simulink model "SimV4"  (R2024b)
settings: Solver=VariableStepAuto  StartTime=0.0  StopTime=30  RelTol=1e-3
model workspace (MAT data in the model file):
  Sig = Simulink.Signal
  Sig.Dimensions = -1
  Sig.DimensionsMode = 'auto'
  Sig.Complexity = 'auto'
  Sig.SampleTime = -1
  Sig.SamplingMode = 'auto'
  Sig.DataType = 'auto'
values from neighbouring files (symbols this model uses):
  CanaryAmplitude = 0.25    [ConfigData.sldd]
  CanaryCarrierFrequency = 20000.0    [ConfigData.sldd]
  CanaryDataRate = 100.0    [ConfigData.sldd]
  DataAmplitude = 0.1    [ConfigData.sldd]
  PreConvolveDownsample = 32.0    [ConfigData.sldd]
  SampleRate = 48000.0    [ConfigData.sldd]
  WalshCodeIndex = 9.0 3.0    [ConfigData.sldd]
undefined symbols (not defined in the file or in its folder): magnitude, WalshCodeCache
libraries: dspfdesign x7, simulink x3, audiosources x2, dspstat3 x2, dspsigops x2, commseqgen3 x2, commchan3 x1, dspsnks4 x1
settings Model: DataDictionary=ConfigData.sldd  SimulationMode=accelerator  PauseTimes=4.5  PacingRate=0.007100  Creator=calum  LastModifiedBy=calum
settings SolverCC: AllowMultiTaskInputOutput=on
settings OptimizationCC: StateBitsets=on  DataBitsets=on  SimCompilerOptimization=on  AccelVerboseBuild=on
settings DebuggingCC: IntegerOverflowMsg=none  IntegerSaturationMsg=none
settings HardwareCC: ProdBitPerLong=64  ProdHWDeviceType=Intel->x86-64 (Linux 64)
settings ModelReferenceCC: UpdateModelReferenceTargets=IfOutOfDate  EnableParallelModelReferenceBuilds=on  ParallelModelReferenceMATLABWorkerInit=Copy Base Workspace
settings SFSimCC: SimCtrlC=off  SimHardwareAcceleration=native
settings RTWCC: GenerateReport=on  Toolchain=GNU gcc/g++ | gmake (64-bit Linux)  BuildConfiguration=Specify  LaunchReport=on
settings GRTTargetCC: OptimizeReductions=on

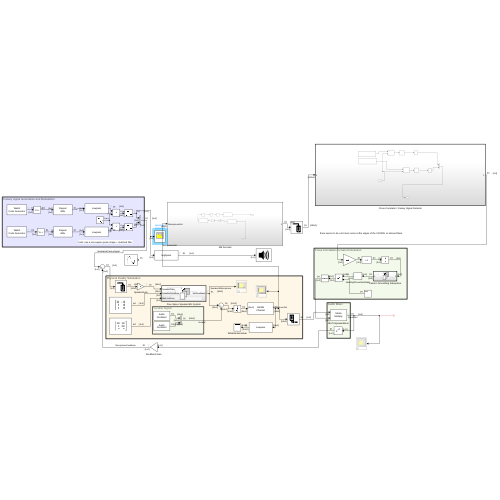
[thumbnail: Simulink's stored preview of the top-level diagram]
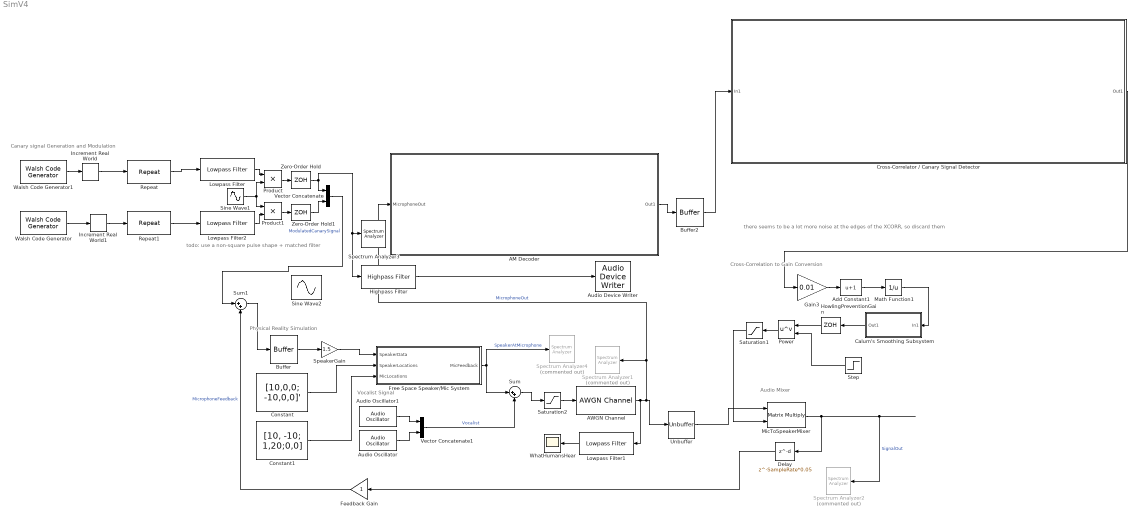
== system SimV4 ==
  note: Canary signal Generation and Modulation
  note: Audio Mixer
  note: Physical Reality Simulation
  note: Vocalist Signal
  note: Cross-Correlation to Gain Conversion
  note: there seems to be a lot more noise at the edges of the XCORR, so discard them
  note: todo: use a non-square pulse shape + matched filter
  "AM Decoder " : Subsystem  Latency=2
  AWGN Channel : commchan3/AWGN Channel  LegacyMode=off  NoiseMethod="Signal to noise ratio  (SNR)"  noiseMode="Signal to noise ratio  (SNR)"  EbNo=10  EsNo=10  SNR=60  BitsPerSymbol=1  SignalPower=1  SamplesPerSymbol=1  SymbolPeriod=1  VarianceSource=Parameter  Variance=1  RandomStream=Global stream  Seed=67  SimulateUsing=Code generation
  Add Constant1 : Bias  Bias=1  SaturateOnIntegerOverflow=off
  Audio Device Writer : dspsnks4/Audio Device Writer  Driver=ALSA  Device=HDA Intel PCH: ALC3254 Analog (hw:0,0)  InheritSampleRate=off  SampleRate=SampleRate  BitDepth=32-bit float  BufferSize=4096  NumBuffers=10  DefaultOutputChannelMapping=on  OutputChannelMapping=1:2  OutputNumUnderrunSamples=off  DriverIdx=8  DeviceWarnFlag=''
  Audio Oscillator : audiosources/Audio Oscillator  FrequencyPort=off  Frequency=200  AmplitudePort=off  Amplitude=DataAmplitude  DCOffsetPort=off  DCOffset=0  PhaseOffset=0  WidthPort=off  Width=1  DutyCyclePort=off  DutyCycle=0.5  SampsPerFrame=64  Fs=SampleRate  OutputDataType=double  SimulateUsing=Code generation
      settings: SignalType=sine
  Audio Oscillator1 : audiosources/Audio Oscillator  FrequencyPort=off  Frequency=400  AmplitudePort=off  Amplitude=DataAmplitude  DCOffsetPort=off  DCOffset=0  PhaseOffset=0  WidthPort=off  Width=1  DutyCyclePort=off  DutyCycle=0.5  SampsPerFrame=64  Fs=SampleRate  OutputDataType=double  SimulateUsing=Code generation
      settings: SignalType=sine
  Buffer : Buffer  OutputFrames=off
  Buffer2 : Buffer  N=ceil(SampleRate/32/CanaryDataRate*32)+10  V=ceil(SampleRate/32/CanaryDataRate*32)+2  OutputFrames=off
  Calum's Smoothing Subsystem : Subsystem  TreatAsAtomicUnit=on
  Constant : Constant  Value="[10,0,0;  -10,0,0]'"
  Constant1 : Constant  Value=[10, -10; 1,20;0,0]
  "Cross-Correlator / Canary Signal Detector " : Subsystem  TreatAsAtomicUnit=on
  Delay : Delay  DelayLength=SampleRate*0.05  InitialCondition=0
  Feedback Gain : Gain
  Free Space Speaker/Mic System : Subsystem  TreatAsAtomicUnit=on
  Gain3 : Gain  Gain=0.01
  Highpass Filter : dspfdesign/Highpass Filter  FilterType=FIR  DesignForMinimumOrder=on  FilterOrder=50  StopbandFrequency=CanaryCarrierFrequency-1000  PassbandFrequency=CanaryCarrierFrequency  StopbandAttenuation=80  PassbandRipple=0.1  SampleRateMode=Specify on dialog  SampleRate=SampleRate  SimulateUsing=Code generation  roundingMode=Floor  coeffsDataTypeStr=fixdt(1,16)
  HowlingPreventionGain : ZeroOrderHold  SampleTime=1/(CanaryDataRate)
  Increment Real World : simulink/Additional Math & Discrete/Additional Math: Increment - Decrement/Increment Real World
  Increment Real World1 : simulink/Additional Math & Discrete/Additional Math: Increment - Decrement/Increment Real World
  Lowpass Filter : dspfdesign/Lowpass Filter  FilterType=IIR  DesignForMinimumOrder=on  FilterOrder=50  PassbandFrequency=CanaryDataRate*2  StopbandFrequency=CanaryDataRate*10  PassbandRipple=0.5  StopbandAttenuation=80  SampleRateMode=Specify on dialog  SampleRate=SampleRate  SimulateUsing=Code generation  roundingMode=Floor  coeffsDataTypeStr=fixdt(1,16)
  Lowpass Filter1 : dspfdesign/Lowpass Filter  FilterType=FIR  DesignForMinimumOrder=on  FilterOrder=50  PassbandFrequency=CanaryCarrierFrequency-8000  StopbandFrequency=CanaryCarrierFrequency-1000  PassbandRipple=0.1  StopbandAttenuation=80  SampleRateMode=Specify on dialog  SampleRate=SampleRate  SimulateUsing=Code generation  roundingMode=Floor  coeffsDataTypeStr=fixdt(1,16)
  Lowpass Filter2 : dspfdesign/Lowpass Filter  FilterType=IIR  DesignForMinimumOrder=on  FilterOrder=50  PassbandFrequency=CanaryDataRate*2  StopbandFrequency=CanaryDataRate*10  PassbandRipple=0.5  StopbandAttenuation=80  SampleRateMode=Specify on dialog  SampleRate=SampleRate  SimulateUsing=Code generation  roundingMode=Floor  coeffsDataTypeStr=fixdt(1,16)
  Math Function1 : Math  Operator=reciprocal
  MicToSpeakerMixer : Product  Multiplication=Matrix(*)
  Power : Math  Operator=pow
  Product : Product
  Product1 : Product
  Repeat : dspsigops/Repeat  FactorSource=Dialog parameter  N=SampleRate/CanaryDataRate  Nmax=16  InputProcessing=Columns as channels (frame based)  RateOptions=Allow multirate processing  ic=0  mode=Unused parameter value
      settings: LibrarySourceBlock=commsequence2/Repeat
  Repeat1 : dspsigops/Repeat  FactorSource=Dialog parameter  N=SampleRate/CanaryDataRate  Nmax=16  InputProcessing=Columns as channels (frame based)  RateOptions=Allow multirate processing  ic=0  mode=Unused parameter value
      settings: LibrarySourceBlock=commsequence2/Repeat
  Saturation1 : Saturate  UpperLimit=1  LowerLimit=0
  Saturation2 : Saturate  UpperLimit=1000  LowerLimit=-1000
  Sine Wave1 : Sin  Amplitude=CanaryAmplitude  Frequency=2*pi*CanaryCarrierFrequency  SampleTime=0
  Sine Wave2 : Sin  Frequency=2*pi*(CanaryCarrierFrequency-1000)  SampleTime=1/SampleRate
  SpeakerGain : Gain  Gain=1.5
  Spectrum Analyzer1 : SpectrumAnalyzer  Commented=on  WindowPosition=[1.000000,38.000000,1920.000000,1003.000000,]  ScopeFrameLocation=window  SampleRateSource=Property  SampleRate=SampleRate  PlotAsTwoSidedSpectrum=off  FrequencyScale=Log  FrequencySpan=Start and stop frequencies  StartFrequency=20  StopFrequency=20e3  YLimits=[-78.74086897,62.76889366]
  Spectrum Analyzer2 : SpectrumAnalyzer  Commented=on  WindowPosition=[1.000000,38.000000,1920.000000,1003.000000,]  ScopeFrameLocation=window  SampleRateSource=Property  SampleRate=SampleRate  PlotAsTwoSidedSpectrum=off  FrequencyScale=Log  FrequencySpan=Start and stop frequencies  StartFrequency=20  StopFrequency=20e3  YLimits=[-81.26361088,68.62221432]
  Spectrum Analyzer3 : SpectrumAnalyzer  WindowPosition=[1.000000,1.000000,1920.000000,1003.000000,]  Visible=on  ScopeFrameLocation=window  Method=Welch  SampleRateSource=Property  SampleRate=SampleRate  PlotAsTwoSidedSpectrum=off  FrequencyScale=Log  FrequencySpan=Start and stop frequencies  StartFrequency=20  StopFrequency=SampleRate/2  YLimits=[-147.26950534,47.28576259]  SelectedToolstripTab=spectrumAnalyzerToolstrip.estimationTab
  Spectrum Analyzer4 : SpectrumAnalyzer  Commented=on  WindowPosition=[1.000000,38.000000,1920.000000,1003.000000,]  ScopeFrameLocation=window  ViewType=Spectrum and spectrogram  SampleRateSource=Property  SampleRate=SampleRate  PlotAsTwoSidedSpectrum=off  FrequencyScale=Log  FrequencySpan=Start and stop frequencies  StartFrequency=20  StopFrequency=20e3  YLimits=[-136.03313301,69.13471038]  ColorLimits=[-136.03313301,69.13471038]
  Step : Step  Time=35  Before=5  After=0  SampleTime=1/(CanaryDataRate)
  Sum : Sum  Inputs=|++
  Sum1 : Sum  Inputs=|++
  Unbuffer : Unbuffer
  Vector Concatenate : Concatenate  Mode=Multidimensional array  ConcatenateDimension=2
  Vector Concatenate1 : Concatenate  Mode=Multidimensional array  ConcatenateDimension=2
  Walsh Code Generator : commseqgen3/Walsh Code Generator  Length=16  Index=WalshCodeIndex(2)  SampleTime=1/CanaryDataRate  SamplesPerFrame=1  OutputDataType=double  SimulateUsing=Code generation
  Walsh Code Generator1 : commseqgen3/Walsh Code Generator  Length=16  Index=WalshCodeIndex(1)  SampleTime=1/CanaryDataRate  SamplesPerFrame=1  OutputDataType=double  SimulateUsing=Code generation
  WhatHumansHear : Scope
  Zero-Order Hold : ZeroOrderHold  SampleTime=1/SampleRate
  Zero-Order Hold1 : ZeroOrderHold  SampleTime=1/SampleRate
  wires:
  Sine Wave1/1 -> Product/2, Product1/1
  Product/1 -> Zero-Order Hold/1
  Zero-Order Hold1/1 -> Vector Concatenate/2
  Product1/1 -> Zero-Order Hold1/1
  Buffer/1 -> SpeakerGain/1
  Walsh Code Generator1/1 -> Increment Real World/1
  AWGN Channel/1 -> "AM Decoder "/1(MicrophoneOut), Spectrum Analyzer1/1, Unbuffer/1, Lowpass Filter1/1  "MicrophoneOut"
  SpeakerGain/1 -> Free Space Speaker/Mic System/1(SpeakerData)
  Constant/1 -> Free Space Speaker/Mic System/2(SpeakerLocations)
  Constant1/1 -> Free Space Speaker/Mic System/3(MicLocations)
  Increment Real World/1 -> Repeat/1
  Increment Real World1/1 -> Repeat1/1
  Audio Oscillator1/1 -> Vector Concatenate1/1
  Audio Oscillator/1 -> Vector Concatenate1/2
  Add Constant1/1 -> Math Function1/1
  Gain3/1 -> Add Constant1/1
  Vector Concatenate1/1 -> Sum/2  "Vocalist"
  Free Space Speaker/Mic System/1(MicFeedback) -> Sum/1, Spectrum Analyzer4/1  "SpeakerAtMicrophone"
  Sum/1 -> Saturation2/1
  Unbuffer/1 -> MicToSpeakerMixer/1
  Math Function1/1 -> Calum's Smoothing Subsystem/1(In1)
  MicToSpeakerMixer/1 -> Spectrum Analyzer2/1, Delay/1  "SignalOut"
  Calum's Smoothing Subsystem/1(Out1) -> HowlingPreventionGain/1
  Sum1/1 -> Buffer/1
  Delay/1 -> Feedback Gain/1
  HowlingPreventionGain/1 -> Power/1
  Step/1 -> Power/2
  Vector Concatenate/1 -> Sum1/1  "ModulatedCanarySignal"
  Power/1 -> Saturation1/1
  Saturation1/1 -> MicToSpeakerMixer/2
  Saturation2/1 -> AWGN Channel/1
  Feedback Gain/1 -> Sum1/2  "MicrophoneFeedback"
  Lowpass Filter1/1 -> WhatHumansHear/1
  "AM Decoder "/1(Out1) -> Buffer2/1
  Buffer2/1 -> "Cross-Correlator / Canary Signal Detector "/1(In1)
  "Cross-Correlator / Canary Signal Detector "/1(Out1) -> Gain3/1
  Lowpass Filter/1 -> Product/1
  Walsh Code Generator/1 -> Increment Real World1/1
  Lowpass Filter2/1 -> Product1/2
  Repeat/1 -> Lowpass Filter/1
  Repeat1/1 -> Lowpass Filter2/1
  Highpass Filter/1 -> Audio Device Writer/1
  Zero-Order Hold/1 -> Vector Concatenate/1, Highpass Filter/1, Spectrum Analyzer3/1

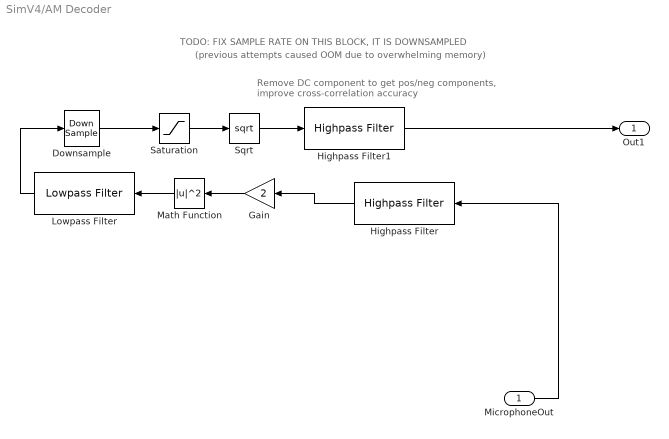
== system SimV4/AM Decoder  ==
  note: (previous attempts caused OOM due to overwhelming memory)
  note: TODO: FIX SAMPLE RATE ON THIS BLOCK, IT IS DOWNSAMPLED
  note: Remove DC component to get pos/neg components,
      | improve cross-correlation accuracy
  MicrophoneOut : Inport
  Downsample : DownSample  N=32
  Gain : Gain  Gain=2
  Highpass Filter : dspfdesign/Highpass Filter  FilterType=FIR  DesignForMinimumOrder=on  FilterOrder=50  StopbandFrequency=CanaryCarrierFrequency-20*CanaryDataRate  PassbandFrequency=CanaryCarrierFrequency-3*CanaryDataRate  StopbandAttenuation=80  PassbandRipple=2  SampleRateMode=Specify on dialog  SampleRate=SampleRate  SimulateUsing=Code generation  roundingMode=Floor  coeffsDataTypeStr=fixdt(1,16)
  Highpass Filter1 : dspfdesign/Highpass Filter  FilterType=FIR  DesignForMinimumOrder=on  FilterOrder=50  StopbandFrequency=5  PassbandFrequency=CanaryDataRate  StopbandAttenuation=80  PassbandRipple=1  SampleRateMode=Specify on dialog  SampleRate=SampleRate  SimulateUsing=Code generation  roundingMode=Floor  coeffsDataTypeStr=fixdt(1,16)
  Lowpass Filter : dspfdesign/Lowpass Filter  FilterType=FIR  DesignForMinimumOrder=on  FilterOrder=50  PassbandFrequency=CanaryDataRate*2  StopbandFrequency=CanaryDataRate*20  PassbandRipple=0.1  StopbandAttenuation=80  SampleRateMode=Specify on dialog  SampleRate=SampleRate  SimulateUsing=Code generation  roundingMode=Floor  coeffsDataTypeStr=fixdt(1,16)
  Math Function : Math  Operator=magnitude^2
  Saturation : Saturate  UpperLimit=inf  LowerLimit=0
  Sqrt : Sqrt
  Out1 : Outport
  wires:
  Gain/1 -> Math Function/1
  Highpass Filter/1 -> Gain/1
  Highpass Filter1/1 -> Out1/1
  Lowpass Filter/1 -> Downsample/1
  Math Function/1 -> Lowpass Filter/1
  Sqrt/1 -> Highpass Filter1/1
  Saturation/1 -> Sqrt/1
  Downsample/1 -> Saturation/1
  MicrophoneOut/1 -> Highpass Filter/1

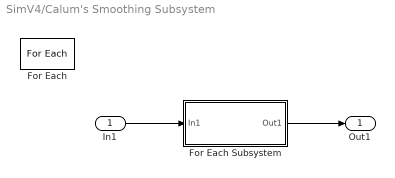
== system SimV4/Calum's Smoothing Subsystem ==
  In1 : Inport  Partition=on  PartitionDimension=1  PartitionWidth=1  PartitionOffset=0
  For Each : ForEach  DisableCoverage=on
  For Each Subsystem : Subsystem  TreatAsAtomicUnit=on
  Out1 : Outport  ConcatenationDimension=1
  wires:
  In1/1 -> For Each Subsystem/1(In1)
  For Each Subsystem/1(Out1) -> Out1/1

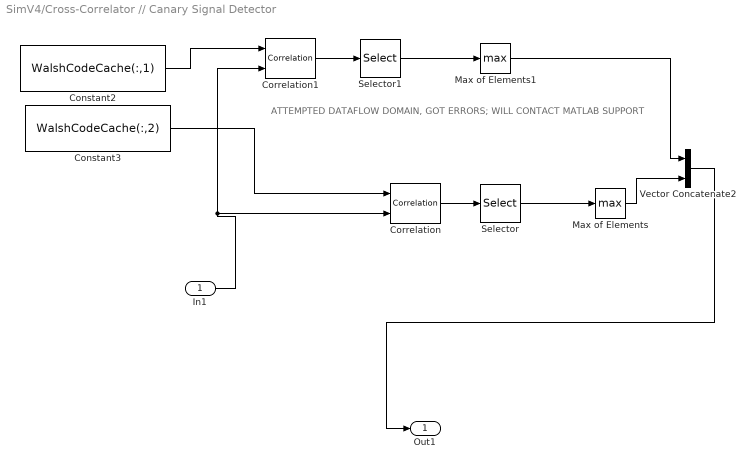
== system SimV4/Cross-Correlator // Canary Signal Detector  ==
  note: ATTEMPTED DATAFLOW DOMAIN, GOT ERRORS; WILL CONTACT MATLAB SUPPORT
  In1 : Inport
  Constant2 : Constant  Value=WalshCodeCache(:,1)  VectorParams1D=off
  Constant3 : Constant  Value=WalshCodeCache(:,2)  VectorParams1D=off
  Correlation : dspstat3/Correlation  domain=Time  roundingMode=Floor  overflowMode=off  outputDataTypeStr=Inherit: Same as accumulator  outputMin=[]  outputMax=[]  outputLastDataTypeStr=Inherit: Same as accumulator
  Correlation1 : dspstat3/Correlation  domain=Fastest  roundingMode=Floor  overflowMode=off  outputDataTypeStr=Inherit: Same as accumulator  outputMin=[]  outputMax=[]  outputLastDataTypeStr=Inherit: Same as accumulator
  Max of Elements : MinMax  Function=max  CollapseMode=Specified dimension
  Max of Elements1 : MinMax  Function=max  CollapseMode=Specified dimension
  Selector : Selector  NumberOfDimensions=2  InputPortWidth=3  IndexOptions=Index vector (dialog),Select all  Indices=[225 : 225+221],1  OutputSizes=1,1
  Selector1 : Selector  NumberOfDimensions=2  InputPortWidth=3  IndexOptions=Index vector (dialog),Select all  Indices=[225 : 225+221],1  OutputSizes=1,1
  Vector Concatenate2 : Concatenate  Mode=Multidimensional array
  Out1 : Outport
  wires:
  Constant2/1 -> Correlation1/1
  Selector/1 -> Max of Elements/1
  Constant3/1 -> Correlation/1
  Max of Elements1/1 -> Vector Concatenate2/1
  Max of Elements/1 -> Vector Concatenate2/2
  Correlation/1 -> Selector/1
  Correlation1/1 -> Selector1/1
  In1/1 -> Correlation/2, Correlation1/2
  Selector1/1 -> Max of Elements1/1
  Vector Concatenate2/1 -> Out1/1

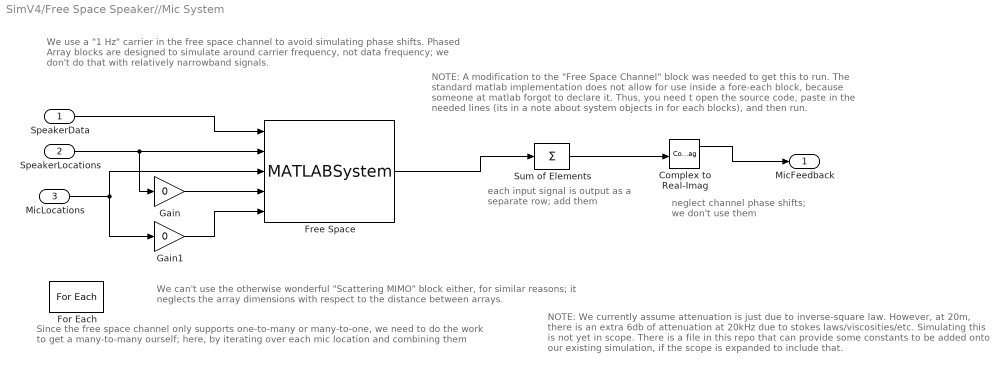
== system SimV4/Free Space Speaker//Mic System ==
  note: NOTE: We currently assume attenuation is just due to inverse-square law.
      | However, at 20m, there is an extra 6db of attenuation at 20kHz due to stokes laws/viscosities/etc.  Simulating this is not yet in scope.  There is a file in this repo that can provide some constants to be added onto our existing simulation, if the scope is expanded to include that.
  note: neglect channel phase
      | shifts; we don't use them
  note: each input signal is output as
      | a separate row; add them
  note: NOTE: A modification to the "Free Space Channel" block was needed to get
      | this to run.  The standard matlab implementation does not allow for use inside a fore-each block, because someone at matlab forgot to declare it.  Thus, you need t open the source code, paste in the needed lines (its in a note about system objects in for each blocks), and then run.
  note: Since the free space channel only supports one-to-many or many-to-one, we need to do the work to get a many-to-many ourself; here, by iterating over each mic location and combining them
  note: We can't use the otherwise wonderful "Scattering MIMO" block either, for similar reasons;
      | it neglects the array dimensions with respect to the distance between arrays.
  note: We use a "1 Hz" carrier in the free space channel to avoid simulating phase shifts.
      | Phased Array blocks are designed to simulate around carrier frequency, not data frequency; we don't do that
      | with relatively narrowband signals.
  SpeakerData : Inport
  SpeakerLocations : Inport  Port=2
  MicLocations : Inport  Port=3  Partition=on  PartitionDimension=2  PartitionWidth=1  PartitionOffset=0
  Complex to Real-Imag : ComplexToRealImag
  For Each : ForEach  DisableCoverage=on
  Free Space : MATLABSystem  System=FreeSpaceCalum  PropagationSpeed=SoundSpeed  OperatingFrequency=0.000001  TwoWayPropagation=off  SampleRateFromInputCheckbox=on  SampleRate=1e6  MaximumDistanceSource=Property  MaximumDistance=10e3  MaximumNumInputSamplesSource=Auto  MaximumNumInputSamples=100  SimulateUsing=Code generation
      settings: LibrarySourceBlock=phasedenvlib/Free Space
      mask Type: FreeSpaceCalum
      mask Display:
      | disp(['Free Space' char(10) 'Channel (Calum''s)']);
      | port_label('input',1,'X');
      | port_label('input',2,'Pos1');
      | port_label('input',3,'Pos2');
      | port_label('input',4,'Vel1');
      | port_label('input',5,'Vel2');
  Gain : Gain  Gain=0
  Gain1 : Gain  Gain=0
  Sum of Elements : Sum  Inputs=+  CollapseMode=Specified dimension  CollapseDim=2
  MicFeedback : Outport  ConcatenationDimension=2
  wires:
  SpeakerData/1 -> Free Space/1
  SpeakerLocations/1 -> Free Space/2, Gain/1
  Free Space/1 -> Sum of Elements/1
  Sum of Elements/1 -> Complex to Real-Imag/1
  Gain/1 -> Free Space/4
  Gain1/1 -> Free Space/5
  MicLocations/1 -> Gain1/1, Free Space/3
  Complex to Real-Imag/1 -> MicFeedback/1

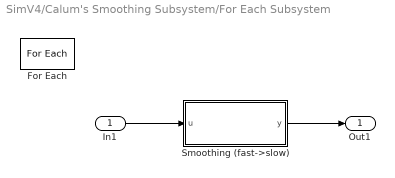
== system SimV4/Calum's Smoothing Subsystem/For Each Subsystem ==
  In1 : Inport  Partition=on  PartitionDimension=2  PartitionWidth=1  PartitionOffset=0
  For Each : ForEach  DisableCoverage=on
  Smoothing (fast->slow) : Subsystem  mask(Smoothing (fast->slow)){nSmooth=floor(SampleRate/CanaryDataRate/PreConvolveDownsample), h1=-1, smoothing0=1}
      mask prompts: nSmooth "physmod:simscape:couplers:SimscapeNetworkCouplersLib:NumberOfSamplesOverWhichToSmooth_MP"; h1 "physmod:simscape:couplers:SimscapeNetworkCouplersLib:PortUDiscreteSampleTimes_MP"; smoothing0 "physmod:simscape:couplers:SimscapeNetworkCouplersLib:InitialOutput_MP"
      mask help: physmod:simscape:couplers:SimscapeNetworkCouplersLib:Smoothingfastslow_MD
      mask Help: web([docroot '/simscape/ref/smoothingfastslow.html'])
      mask DialogControl nSmooth Prompt: Number of samples over which to smooth
      mask DialogControl h1 Prompt: Port u discrete sample time (s)
      mask DialogControl smoothing0 Prompt: Initial output
  Out1 : Outport  ConcatenationDimension=2
  wires:
  In1/1 -> Smoothing (fast->slow)/1(u)
  Smoothing (fast->slow)/1(y) -> Out1/1

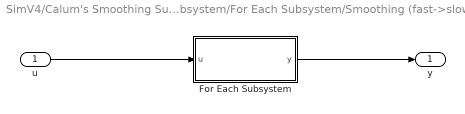
== system SimV4/Calum's Smoothing Subsystem/For Each Subsystem/Smoothing (fast->slow) ==
  u : Inport
  For Each Subsystem : Subsystem  TreatAsAtomicUnit=on
  y : Outport
  wires:
  For Each Subsystem/1(y) -> y/1
  u/1 -> For Each Subsystem/1(u)

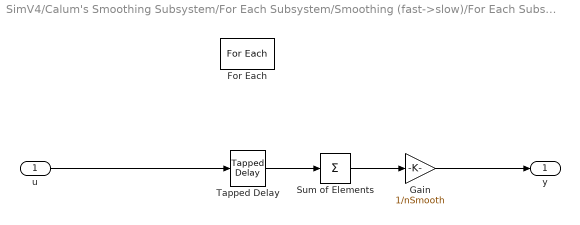
== system SimV4/Calum's Smoothing Subsystem/For Each Subsystem/Smoothing (fast->slow)/For Each Subsystem ==
  u : Inport  Partition=on  PartitionDimension=1  PartitionWidth=1  PartitionOffset=0
  For Each : ForEach  DisableCoverage=on
  Gain : Gain  Gain=1/nSmooth
  Sum of Elements : Sum  Inputs=+
  Tapped Delay : simulink/Discrete/Tapped Delay  vinit=mean(smoothing0)  samptime=h1  NumDelays=nSmooth  DelayOrder=Oldest  includeCurrent=off
  y : Outport  ConcatenationDimension=1
  wires:
  u/1 -> Tapped Delay/1
  Sum of Elements/1 -> Gain/1
  Tapped Delay/1 -> Sum of Elements/1
  Gain/1 -> y/1
